simulink model "Final_PEM_Model"  (R2024a)
settings: Solver=ode4  StartTime=0.0  StopTime=10  FixedStep=10e-6  RelTol=1e-3
libraries: spsParallelRLCBranchLib x8, spsVoltageMeasurementLib x4, spsDCVoltageSourceLib x2, spsMeanLib x2, spsCurrentMeasurementLib x1, spsDiodeLib x1, sps_lib x1
settings Model: Creator=ADMIN  LastModifiedBy=ADMIN

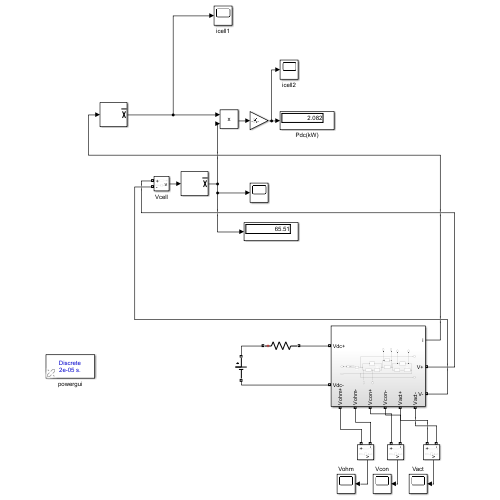
[thumbnail: Simulink's stored preview of the top-level diagram]
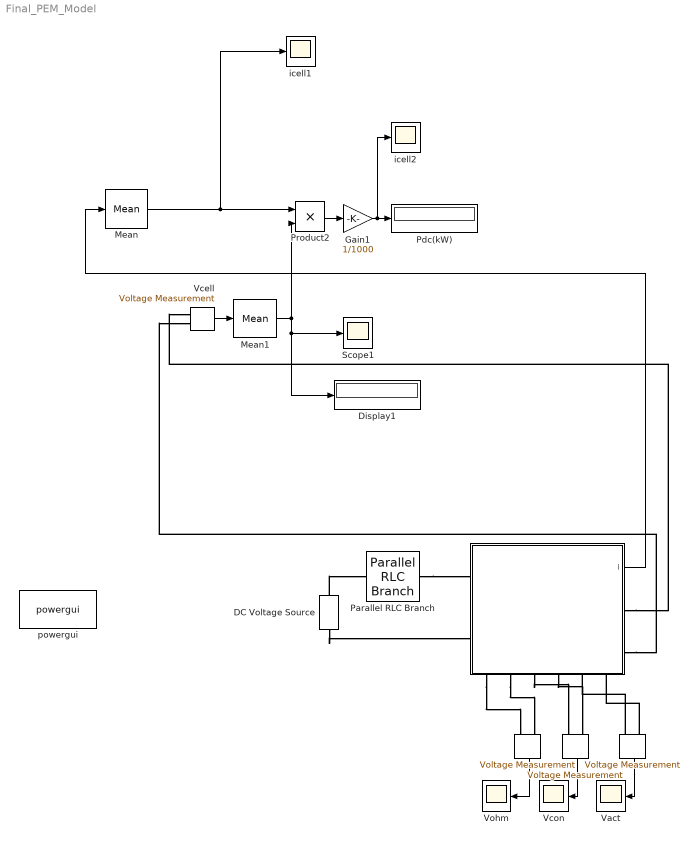
== system Final_PEM_Model ==
  " " : spsVoltageMeasurementLib/Voltage Measurement  PhasorSimulation=off  OutputType=Complex  PSBequivalent=0
  "   " : spsVoltageMeasurementLib/Voltage Measurement  PhasorSimulation=off  OutputType=Complex  PSBequivalent=0
  "      " : spsVoltageMeasurementLib/Voltage Measurement  PhasorSimulation=off  OutputType=Complex  PSBequivalent=0
  "                          " : Subsystem
      settings: PortSchema="{\"entries\":[{\"content\":{\"sides\":[{\"content\":{\"connectorIds\":[\"LConn1\",\"LConn2\"]},\"type\":\"ConnectorPlacement.EquallySpacedRectSide\",\"uuid\":\"5295d51d-6d5e-4747-a193-168dafaf2bb6\"},{\"content\":{\"connectorIds\":[\"Out1\",\"RConn1\",\"RConn2\"],\"side\":\"RIGHT\"},\"type\":\"ConnectorPlacement.EquallySpacedRectSide\",\"uuid\":\"4c99502c-1d19-44cf-9b72-2f4631be0f61\"},{\"content\":{\"side\":\"TOP\"},\"type\":\"ConnectorPlacement.EquallySpacedRectSide\",\"uuid\":\"0c355641-6deb-4edf-9744-e746ac7c044e\"},{\"content\":{\"connectorIds\":[\"RConn3\",\"RConn4\",\"RConn5\",\"RConn6\",\"RConn7\",\"RConn8\"],\"side\":\"BOTTOM\"},\"type\":\"ConnectorPlacement.EquallySpacedRectSide\",\"uuid\":\"f5d53cca-348f-4a40-9b5d-09adf7770e7b\"}]},\"type\":\"ConnectorPlacement.EquallySpacedConnector\",\"uuid\":\"73017685-9e7a-4c5d-9365-d4c2efcd3dff\"}],\"packageUris\":[\"http://schema.mathworks.com/mf0/Connector/R2020b\"],\"version\":\"1.0\"}"
  DC Voltage Source : spsDCVoltageSourceLib/DC Voltage Source  Amplitude=100  Measurements=None
  Display1 : Display
      settings: Format=bank
  Gain1 : Gain  Gain=1/1000
  Mean : spsMeanLib/Mean  Freq=60  Vinit=0  Ts=50e-6
  Mean1 : spsMeanLib/Mean  Freq=60  Vinit=0  Ts=50e-6
  Parallel RLC Branch : spsParallelRLCBranchLib/Parallel RLC Branch  LConnTagsString=a  RConnTagsString=__new0  BranchType=R  Resistance=1  Inductance=1e-3  SetiL0=off  InitialCurrent=0  Capacitance=1e-6  Setx0=off  InitialVoltage=0  Measurements=None
  Pdc(kW) : Display
  Product2 : Product
  Scope1 : Scope
  Vact : Scope
  Vcell : spsVoltageMeasurementLib/Voltage Measurement  PhasorSimulation=off  OutputType=Complex  PSBequivalent=0
  Vcon : Scope
  Vohm : Scope
  icell1 : Scope
  icell2 : Scope
  powergui : sps_lib/powergui  Priority=1  SimulationMode=Discrete  SampleTime=20e-6  frequency=60  Iterations=50  frequencyindice=0  Pbase=100e6  ErrMax=1e-4  UnitsV=kV  UnitsW=MW  buscounter=0  FunctionMessages=off  echomessages=off  EnableUseOfTLC=off  CurrentSourceSwitches=off  DisableSnubberDevices=off  DisableRonSwitches=off  DisableVfSwitches=off  DisplayEquations=off  AutomaticDiscreteSolvers=off  SolverType=Tustin/Backward Euler (TBE)  Interpol=off  ExternalGateDelay=off  methode=off  Ts=100  x0status=blocks  SPID=on  SwTol=0  HookPort=off  NonlinearTolerance=1e-4  nMaxIteration=100  ContinueOnMaxIteration=off  RestoreLinks=warning  ResistiveCurrentMeasurement=off  Frange=[0:2:500]  Ylog=off  Xlog=on  ShowGrid=off  save=off  variable=ZData  structure=0  ZoomFFT=off  StartTime=0.0  cycles=1  DisplayStyle=1  fundamental=60  FreqAxis=off  MaxFrequency=1000  frequencyindicesteady=1  RmsSteady=1  display=off
  wires:
  " "/1 -> Vcon/1
  "   "/1 -> Vact/1
  "      "/1 -> Vohm/1
  Mean1/1 -> Scope1/1, Display1/1, Product2/2
  Vcell/1 -> Mean1/1
  "                          "/1(i) -> Mean/1
  Mean/1 -> Product2/1, icell1/1
  Product2/1 -> Gain1/1
  Gain1/1 -> icell2/1, Pdc(kW)/1
  connections:
  "                          "/RConn2 -- Vcell/LConn2
  "                          "/RConn1 -- Vcell/LConn1
  "   "/LConn1 -- "                          "/RConn7
  "                          "/RConn5 -- " "/LConn1
  "                          "/RConn4 -- "      "/LConn2
  "                          "/RConn6 -- " "/LConn2
  "   "/LConn2 -- "                          "/RConn8
  "                          "/RConn3 -- "      "/LConn1
  Parallel RLC Branch/RConn1 -- "                          "/LConn1
  DC Voltage Source/LConn1 -- "                          "/LConn2
  DC Voltage Source/RConn1 -- Parallel RLC Branch/LConn1

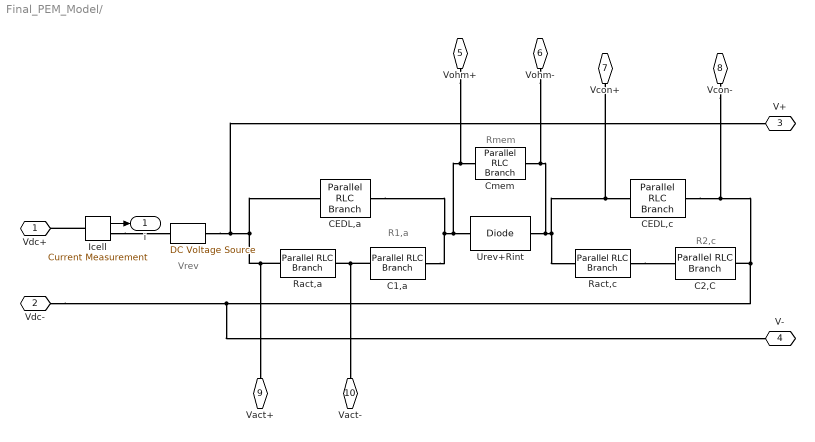
== system Final_PEM_Model/                           ==
  note: Vrev
  note: R1,a
  note: R2,c
  note: Rmem
  " " : spsDCVoltageSourceLib/DC Voltage Source  Amplitude=2.71  Measurements=None
  C1,a : spsParallelRLCBranchLib/Parallel RLC Branch  LConnTagsString=a  RConnTagsString=__new0  BranchType=RC  Resistance=0.01  Inductance=1e-3  SetiL0=off  InitialCurrent=0  Capacitance=100  Setx0=off  InitialVoltage=0  Measurements=None
  C2,C : spsParallelRLCBranchLib/Parallel RLC Branch  LConnTagsString=a  RConnTagsString=__new0  BranchType=RC  Resistance=0.005  Inductance=1e-3  SetiL0=off  InitialCurrent=0  Capacitance=100  Setx0=off  InitialVoltage=0  Measurements=None
  CEDL,a : spsParallelRLCBranchLib/Parallel RLC Branch  LConnTagsString=a  RConnTagsString=__new0  BranchType=C  Resistance=1  Inductance=1e-3  SetiL0=off  InitialCurrent=0  Capacitance=1.93  Setx0=off  InitialVoltage=0  Measurements=None
  CEDL,c : spsParallelRLCBranchLib/Parallel RLC Branch  LConnTagsString=a  RConnTagsString=__new0  BranchType=C  Resistance=1  Inductance=1e-3  SetiL0=off  InitialCurrent=0  Capacitance=1.93  Setx0=off  InitialVoltage=0  Measurements=None
  Cmem : spsParallelRLCBranchLib/Parallel RLC Branch  LConnTagsString=a  RConnTagsString=__new0  BranchType=RC  Resistance=0.1025  Inductance=1e-3  SetiL0=off  InitialCurrent=0  Capacitance=0.1  Setx0=off  InitialVoltage=0  Measurements=None
  Icell : spsCurrentMeasurementLib/Current Measurement  PhasorSimulation=off  OutputType=Complex  PSBequivalent=0
  Ract,a : spsParallelRLCBranchLib/Parallel RLC Branch  LConnTagsString=a  RConnTagsString=__new0  BranchType=R  Resistance=1  Inductance=1e-3  SetiL0=off  InitialCurrent=0  Capacitance=1e-6  Setx0=off  InitialVoltage=0  Measurements=None
  Ract,c : spsParallelRLCBranchLib/Parallel RLC Branch  LConnTagsString=a  RConnTagsString=__new0  BranchType=R  Resistance=1  Inductance=1e-3  SetiL0=off  InitialCurrent=0  Capacitance=1e-6  Setx0=off  InitialVoltage=0  Measurements=None
  Urev+Rint : spsDiodeLib/Diode  Ron=0.0001  Lon=0  Vf=1.48  IC=0  UseSnubber=0  Rs=0  Cs=0  Measurements=off
  Vdc+ : PMIOPort  Side=Left
  Vdc- : PMIOPort  Port=2  Side=Left
  V+ : PMIOPort  Port=3  Side=Right
  V- : PMIOPort  Port=4  Side=Right
  Vohm+ : PMIOPort  Port=5  Side=Right
  Vohm- : PMIOPort  Port=6  Side=Right
  Vcon+ : PMIOPort  Port=7  Side=Right
  Vcon- : PMIOPort  Port=8  Side=Right
  Vact+ : PMIOPort  Port=9  Side=Right
  Vact- : PMIOPort  Port=10  Side=Right
  i : Outport
  wires:
  Icell/1 -> i/1
  connections:
  C1,a/RConn1 -- CEDL,a/RConn1 -- Vohm+/RConn1 -- Cmem/LConn1 -- Urev+Rint/LConn1
  Urev+Rint/RConn1 -- Cmem/RConn1 -- Vohm-/RConn1 -- Ract,c/LConn1 -- CEDL,c/LConn1 -- Vcon+/RConn1
  Icell/LConn1 -- Vdc+/RConn1
  C1,a/LConn1 -- Vact-/RConn1 -- Ract,a/RConn1
  CEDL,c/RConn1 -- Vcon-/RConn1 -- V-/RConn1 -- Vdc-/RConn1 -- C2,C/RConn1
  Ract,a/LConn1 -- Vact+/RConn1 -- V+/RConn1 -- " "/LConn1 -- CEDL,a/LConn1
  Icell/RConn1 -- " "/RConn1
  Ract,c/RConn1 -- C2,C/LConn1
